simulink model "velocity_plausibility"  (R2024b)
settings: Solver=FixedStepAuto  StartTime=0.0  StopTime=20  FixedStep=0.1  RelTol=1e-3  EnableMultiTasking=on
settings Model: ExtModeTrigDuration=2  Creator=aayan  LastModifiedBy=aayan
settings SolverCC: AutoInsertRateTranBlk=on
settings OptimizationCC: EnhancedBackFolding=on  PassReuseOutputArgsAs=Individual arguments  ZeroExternalMemoryAtStartup=off  ZeroInternalMemoryAtStartup=off  MaxStackSize=64  OptimizeBlockOrder=speed  DifferentSizesBufferReuse=on  OptimizationCustomize=off  EfficientTunableParamExpr=on
settings DebuggingCC: ParameterTunabilityLossMsg=error
settings HardwareCC: ProdBitPerInt=16  ProdBitPerPointer=16  ProdBitPerSizeT=16  ProdBitPerPtrDiffT=16  ProdLargestAtomicFloat=None  ProdWordSize=8  ProdHWDeviceType=Atmel->AVR
settings SFSimCC: MATLABDynamicMemAlloc=off
settings RTWCC: Description=Embedded Coder  SystemTargetFile=ert.tlc  HardwareBoard=Arduino Uno  GenCodeOnly=on  TemplateMakefile=ert_default_tmf  Toolchain=Arduino AVR  BuildConfiguration=Faster Runs
settings CodeAppCC: ForceParamTrailComments=on  IgnoreCustomStorageClasses=off  OperatorAnnotations=on  SimulinkDataObjDesc=on  SFDataObjDesc=on  InsertBlockDesc=on
settings ERTTargetCC: SupportVariableSizeSignals=on  ExtModeTransport=3  ExtModeStaticAlloc=on  ExtModeAutomaticAllocSize=off  ExtModeStaticAllocSize=250  ExtModeMexFile=ext_xcp  ExtModeIntrfLevel=Level2 - Open  InlinedParameterPlacement=Hierarchical
settings ConfigComp: CovEnable=on  RecordCoverage=on  CovMetricSettings=dcmwe  CovModelRefEnable=on

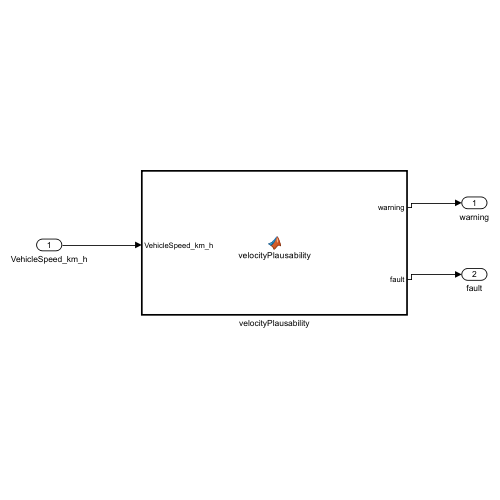
[thumbnail: Simulink's stored preview of the top-level diagram]
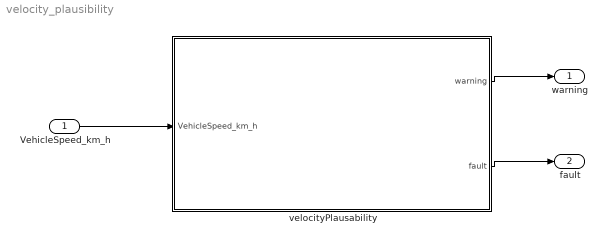
== system velocity_plausibility ==
  VehicleSpeed_km_h : Inport  OutDataTypeStr=single
  velocityPlausability : MATLAB Function  TreatAsAtomicUnit=on
  warning : Outport
  fault : Outport  Port=2
  wires:
  velocityPlausability/1(warning) -> warning/1
  velocityPlausability/2(fault) -> fault/1
  VehicleSpeed_km_h/1 -> velocityPlausability/1(VehicleSpeed_km_h)

== matlab function velocity_plausibility/velocityPlausability ==
  data: VehicleSpeed_km_h input; warning output; fault output
function [warning, fault] = velocityPlausability(VehicleSpeed_km_h)
% initialization
warning = boolean(0);
fault = boolean(0);

if (VehicleSpeed_km_h > 240|| VehicleSpeed_km_h < -60 )
    warning = boolean(1);
    fault = boolean(1);
end
